simulink model "simulink_controller"  (R2019b)
settings: Solver=VariableStepAuto  StartTime=0.0  StopTime=10.0  RelTol=1e-3
libraries: cstblocks x1
settings Model: Creator=Gautam Gupta  LastModifiedBy=Gautam Gupta

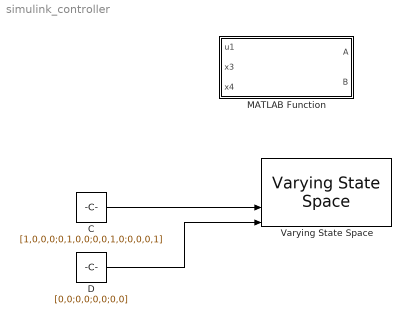
== system simulink_controller ==
  C : Constant  Value=[1,0,0,0;0,1,0,0;0,0,1,0;0,0,0,1]
  D : Constant  Value=[0,0;0,0;0,0;0,0]
  MATLAB Function : MATLAB Function  TreatAsAtomicUnit=on
  Varying State Space : cstblocks/Linear Parameter Varying/Varying State Space  x0=0  xNames=''  OutputX=on  OutputDX=on
      settings: SourceProductName=Control System Toolbox
  wires:
  C/1 -> Varying State Space/4
  D/1 -> Varying State Space/5

== matlab function simulink_controller/MATLAB Function ==
  data: u1 input; A output; x3 input; x4 input; B output
function [A, B] = linearization(u1, x3, x4)
    %Constants
    C = 1/2.551;
%     Q = [1, 0;
%         0, 1];
%     R = [1, 0;
%         0, 1];

    %Linearized state space matrices - 2 inputs, 4 outputs
    A = [0, 0, (-u1*sin(x3)), 0;
                    0, 0, (u1*cos(x3)), 0;
                    0, 0, 0, u1*C*(sec(x4)^2);
                    0, 0, 0, 0];
    B = [cos(x3), 0;
        sin(x3), 0;
        C*tan(x4), 0;
        0, 1];
